simulink model "Acceleration_test"  (R2023b)
settings: Solver=FixedStepAuto  StartTime=0.0  StopTime=30.0  FixedStep=1e-3  RelTol=1e-3  EnableMultiTasking=on
libraries: dspstat3 x3, frdmk64flib x1
settings Model: ExtModeTrigDuration=5  Creator=bardiased  LastModifiedBy=bardiased
settings OptimizationCC: EnhancedBackFolding=on  PassReuseOutputArgsAs=Individual arguments  ZeroExternalMemoryAtStartup=off  ZeroInternalMemoryAtStartup=off  MaxStackSize=64  OptimizeBlockOrder=speed  DifferentSizesBufferReuse=on  OptimizationCustomize=off  EfficientTunableParamExpr=on
settings DebuggingCC: ParameterTunabilityLossMsg=error
settings HardwareCC: ProdBitPerPointer=32  ProdBitPerSizeT=32  ProdBitPerPtrDiffT=32  ProdLargestAtomicInteger=Long  ProdLargestAtomicFloat=Double  ProdWordSize=32  ProdHWDeviceType=ARM Compatible->ARM Cortex
settings SFSimCC: MATLABDynamicMemAlloc=off
settings RTWCC: Description=Embedded Coder  SystemTargetFile=ert.tlc  HardwareBoard=NXP FRDM-K64F  TLCOptions="-aInlineSetEventsForThisBaseRateFcn=TLC_FALSE -aSuppressMultiTaskScheduler=TLC_FALSE  -aRateBasedStepFcn=0"  TemplateMakefile=ert_default_tmf  Toolchain=GNU Tools for ARM Embedded Processors
settings CodeAppCC: ForceParamTrailComments=on  IgnoreCustomStorageClasses=off  OperatorAnnotations=on  SimulinkDataObjDesc=on  SFDataObjDesc=on  InsertBlockDesc=on
settings ERTTargetCC: ExtModeTransport=4  ExtModeMexFile=sendToCommService

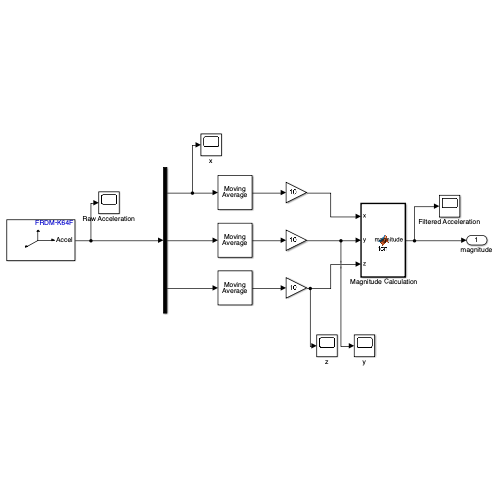
[thumbnail: Simulink's stored preview of the top-level diagram]
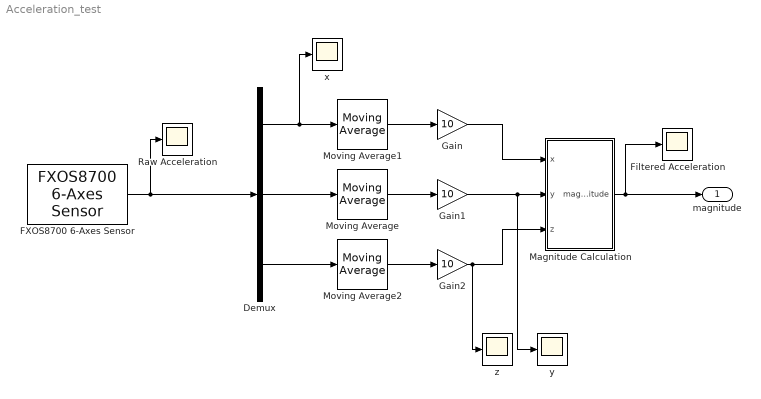
== system Acceleration_test ==
  " Magnitude Calculation" : MATLAB Function  TreatAsAtomicUnit=on
  Demux : Demux  Outputs=3
  FXOS8700 6-Axes Sensor : frdmk64flib/FXOS8700 6-Axes Sensor  Activesensor=Accelerometer only  ODR=800Hz  HybridODR=400Hz  Accelfullrange=-4g to +4g  SampleTime=-1
  Filtered Acceleration : Scope
  Gain : Gain  Gain=10
  Gain1 : Gain  Gain=10
  Gain2 : Gain  Gain=10
  Moving Average : dspstat3/Moving Average  Method=Sliding window  ForgettingFactorPort=off  SpecifyWindowLength=on  WindowLength=4  OverlapLength=3  AllowArbitraryInputLength=off  ForgettingFactor=0.9  SimulateUsing=Code generation
  Moving Average1 : dspstat3/Moving Average  Method=Sliding window  ForgettingFactorPort=off  SpecifyWindowLength=on  WindowLength=4  OverlapLength=3  AllowArbitraryInputLength=off  ForgettingFactor=0.9  SimulateUsing=Code generation
  Moving Average2 : dspstat3/Moving Average  Method=Sliding window  ForgettingFactorPort=off  SpecifyWindowLength=on  WindowLength=4  OverlapLength=3  AllowArbitraryInputLength=off  ForgettingFactor=0.9  SimulateUsing=Code generation
  Raw Acceleration : Scope
  x : Scope
  y : Scope
  z : Scope
  magnitude : Outport
  wires:
  Demux/2 -> Moving Average/1
  " Magnitude Calculation"/1(magnitude) -> Filtered Acceleration/1, magnitude/1
  Demux/3 -> Moving Average2/1
  Gain2/1 -> z/1, " Magnitude Calculation"/3(z)
  Gain/1 -> " Magnitude Calculation"/1(x)
  Moving Average1/1 -> Gain/1
  Demux/1 -> x/1, Moving Average1/1
  Gain1/1 -> y/1, " Magnitude Calculation"/2(y)
  Moving Average/1 -> Gain1/1
  FXOS8700 6-Axes Sensor/1 -> Raw Acceleration/1, Demux/1
  Moving Average2/1 -> Gain2/1

== matlab function Acceleration_test/ Magnitude Calculation ==
  data: magnitude output; x input; y input; z input
function magnitude = fcn(x, y, z)
    magnitude = sqrt(x.^2 + y.^2 + z.^2);
end
